simulink model "model1"  (R2023a)
settings: Solver=VariableStepAuto  StartTime=0.0  StopTime=row/100  RelTol=1e-3
values from neighbouring files (symbols this model uses):
  data = load(input_data)    [F1.m]    (also in F1Sy.m; F1Vexp2V.m; F1Vexp2V_SexpS.m; F1Vexp2V_SexpS_ssr.m)
  R = A(2)    [F1.m]    (also in F1Sy.m; F1Vexp2V.m; F1Vexp2V_SexpS.m; F1Vexp2V_SexpS_ssr_all.m = input_parameters(2))
settings Model: Creator=test  LastModifiedBy=test

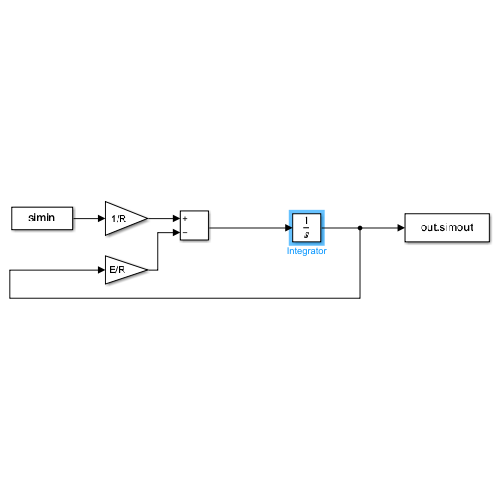
[thumbnail: Simulink's stored preview of the top-level diagram]
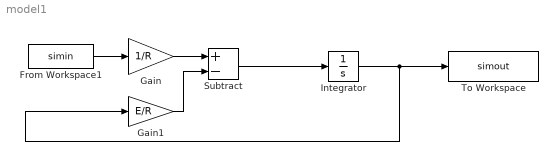
== system model1 ==
  From Workspace1 : FromWorkspace  VariableName=simin
  Gain : Gain  Gain=1/R
  Gain1 : Gain  Gain=E/R
  Integrator : Integrator  InitialCondition=data(1,3)
  Subtract : Sum  Inputs=+-
  To Workspace : ToWorkspace  VariableName=simout  SaveFormat=Timeseries  SampleTime=0.01
  wires:
  Gain/1 -> Subtract/1
  Gain1/1 -> Subtract/2
  Integrator/1 -> To Workspace/1, Gain1/1
  From Workspace1/1 -> Gain/1
  Subtract/1 -> Integrator/1
